simulink model "chap8_2sim"  (Simulink 8.1)
settings: Solver=ode45  StartTime=0.0  StopTime=80  RelTol=1e-3
settings Model: Creator=Administrator  LastModifiedBy=Administrator
settings DataIOCC: InspectSignalLogs=on  SignalLoggingName=sigsOut
settings OptimizationCC: ExpressionDepthLimit=128  InitFltsAndDblsToZero=on
settings DebuggingCC: SaveWithParameterizedLinksMsg=none  SignalResolutionControl=TryResolveAllWithWarning  SolverPrmCheckMsg=none  MultiTaskDSMMsg=warning  MultiTaskCondExecSysMsg=none  StrictBusMsg=None
settings HardwareCC: TargetUnknown=on
settings RTWCC: IncludeERTFirstTime=on
settings GRTTargetCC: TargetFcnLib=ansi_tfl_tmw.mat

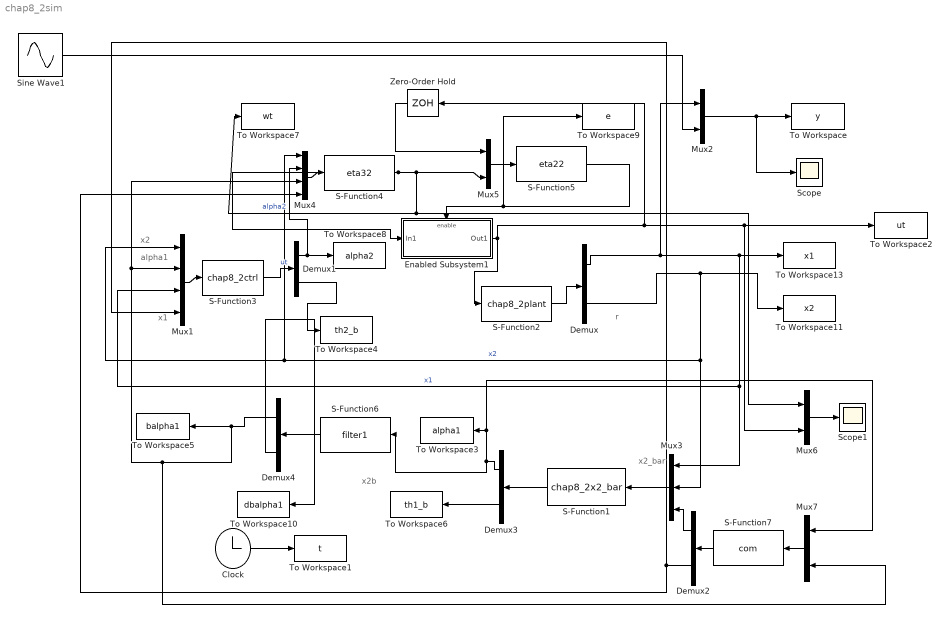
== system chap8_2sim ==
  note: x2
  note: alpha1
  note: x1
  note: x2b
  note: r
  note: x2_bar
  Clock : Clock
  Demux{,1..4} (5 alike) : Demux  Outputs=2
  Enabled Subsystem1 : Subsystem  TreatAsAtomicUnit=on
  Mux1 : Mux
  Mux{2,5..7} (4 alike) : Mux  Inputs=2
  Mux3 : Mux  Inputs=3
  Mux4 : Mux
  S-Function1 : S-Function  FunctionName=chap8_2x2_bar  EnableBusSupport=off
  S-Function2 : S-Function  FunctionName=chap8_2plant  EnableBusSupport=off
  S-Function3 : S-Function  FunctionName=chap8_2ctrl  EnableBusSupport=off
  S-Function4 : S-Function  FunctionName=eta32  EnableBusSupport=off
  S-Function5 : S-Function  FunctionName=eta22  EnableBusSupport=off
  S-Function6 : S-Function  FunctionName=filter1  EnableBusSupport=off
  S-Function7 : S-Function  FunctionName=com  EnableBusSupport=off
  Scope : Scope
  Scope1 : Scope
  Sine Wave1 : Sin  Frequency=0.5  SampleTime=0
  To Workspace : ToWorkspace  VariableName=y  SampleTime=-1
  To Workspace1 : ToWorkspace  VariableName=t  SampleTime=-1
  To Workspace10 : ToWorkspace  VariableName=dbalpha1  SampleTime=-1
  To Workspace11 : ToWorkspace  VariableName=x2  SampleTime=-1
  To Workspace13 : ToWorkspace  VariableName=x1  SampleTime=-1
  To Workspace2 : ToWorkspace  VariableName=ut  SampleTime=-1
  To Workspace3 : ToWorkspace  VariableName=alpha1  SampleTime=-1
  To Workspace4 : ToWorkspace  VariableName=th2_b  SampleTime=-1
  To Workspace5 : ToWorkspace  VariableName=balpha1  SampleTime=-1
  To Workspace6 : ToWorkspace  VariableName=th1_b  SampleTime=-1
  To Workspace7 : ToWorkspace  VariableName=wt  SampleTime=-1
  To Workspace8 : ToWorkspace  VariableName=alpha2  SampleTime=-1
  To Workspace9 : ToWorkspace  VariableName=e  SampleTime=-1
  Zero-Order Hold : ZeroOrderHold
  wires:
  Clock/1 -> To Workspace1/1
  Mux1/1 -> S-Function3/1
  S-Function2/1 -> Demux/1
  Demux/1 -> Mux1/3, Mux3/1, To Workspace13/1, Mux2/1  "x1"
  Demux/2 -> Mux4/1, Mux1/1, Mux3/2, To Workspace11/1  "x2"
  S-Function3/1 -> Demux1/1  "ut"
  S-Function1/1 -> Demux3/1
  Demux3/1 -> Mux7/1, To Workspace3/1, S-Function6/1
  Demux3/2 -> To Workspace6/1
  Mux3/1 -> S-Function1/1
  Demux1/2 -> To Workspace4/1
  Demux1/1 -> Mux4/2, To Workspace8/1  "alpha2"
  Mux2/1 -> Scope/1, To Workspace/1
  Mux4/1 -> S-Function4/1
  S-Function4/1 -> Enabled Subsystem1/1(In1), To Workspace7/1, Mux6/1, Mux5/2
  Enabled Subsystem1/1(Out1) -> S-Function2/1, Zero-Order Hold/1, Mux6/2, To Workspace2/1
  S-Function5/1 -> To Workspace9/1, Enabled Subsystem1/Enable
  Mux5/1 -> S-Function5/1
  Zero-Order Hold/1 -> Mux5/1
  Mux6/1 -> Scope1/1
  Sine Wave1/1 -> Mux2/2
  Mux7/1 -> S-Function7/1
  S-Function7/1 -> Demux2/1
  Demux2/1 -> Mux3/3
  Demux2/2 -> Mux4/4, Mux1/4
  S-Function6/1 -> Demux4/1
  Demux4/1 -> Mux7/2, Mux4/3, Mux1/2, To Workspace5/1
  Demux4/2 -> To Workspace10/1

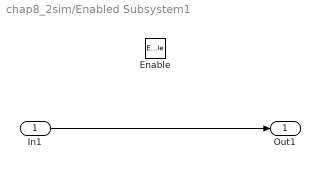
== system chap8_2sim/Enabled Subsystem1 ==
  In1 : Inport
  Enable : EnablePort
  Out1 : Outport
  wires:
  In1/1 -> Out1/1
